simulink model "Seyfi_Ahmadi_Project4"  (R2018b)
settings: Solver=VariableStepAuto  StartTime=0.0  StopTime=50  RelTol=1e-3
settings Model: Creator=DearUser  LastModifiedBy=DearUser

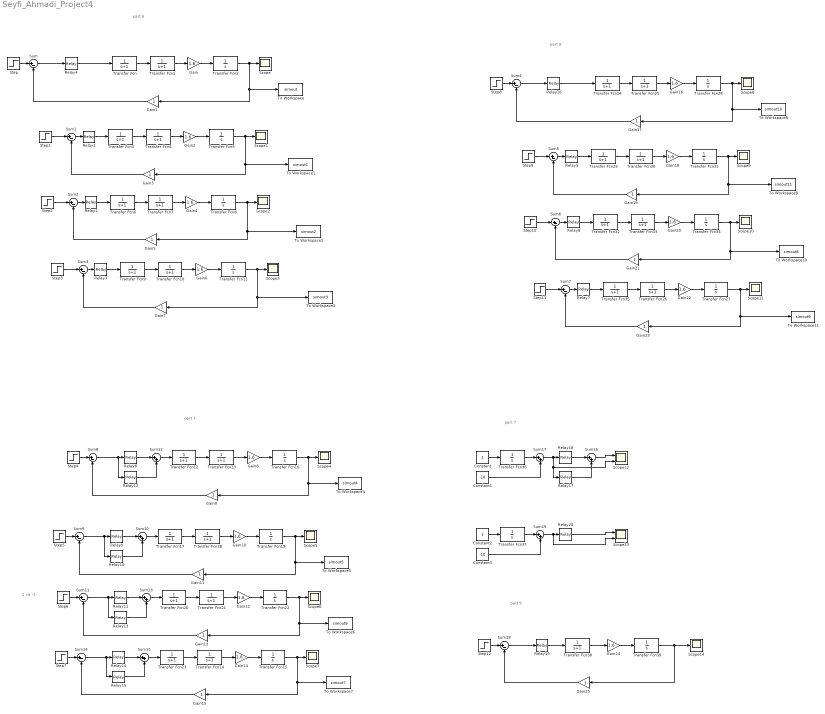
== system Seyfi_Ahmadi_Project4 ==
  note: 1 va -1
  note: part 6
  note: part 7
  note: part 8
  note: part 7
  note: part 9
  Constant : Constant
  Constant1 : Constant  Value=-10
  Constant2 : Constant
  Constant3 : Constant  Value=-10
  Gain{,2,4,6,8,10,12,14,16,18,20,22,24} (13 alike) : Gain  Gain=1.6
  Gain{1,3,5,7,9,11,13,15,17,19,21,23,25} (13 alike) : Gain
  Relay{1..3,7} (4 alike) : Relay  OnSwitchValue=0  OffSwitchValue=0  OnOutputValue=5  OffOutputValue=-5
  Relay10 : Relay  OnSwitchValue=-1.5  OffSwitchValue=-2  OnOutputValue=5  OffOutputValue=-5
  Relay11 : Relay  OnSwitchValue=1  OffSwitchValue=0  OnOutputValue=2.5  OffOutputValue=-2.5
  Relay12 : Relay  OnSwitchValue=0  OffSwitchValue=0  OnOutputValue=2.5  OffOutputValue=-2.5
  Relay13 : Relay  OnSwitchValue=-1  OffSwitchValue=-2.5  OnOutputValue=2.5  OffOutputValue=-2.5
  Relay14 : Relay  OnSwitchValue=2.5  OffSwitchValue=0  OnOutputValue=2.5  OffOutputValue=-2.5
  Relay15 : Relay  OnSwitchValue=-2.5  OffSwitchValue=-4  OnOutputValue=2.5  OffOutputValue=-2.5
  Relay16 : Relay  OnSwitchValue=5  OffSwitchValue=-5  OnOutputValue=3  OffOutputValue=-3
  Relay17 : Relay  OnSwitchValue=-1.5  OffSwitchValue=-3  OnOutputValue=2.5  OffOutputValue=-2.5
  Relay18 : Relay  OnSwitchValue=1.5  OffSwitchValue=0  OnOutputValue=2.5  OffOutputValue=-2.5
  Relay19 : Relay  OnSwitchValue=5  OffSwitchValue=-5  OnOutputValue=5  OffOutputValue=-5
  Relay20 : Relay  OnSwitchValue=0  OffSwitchValue=0  OnOutputValue=2.5  OffOutputValue=-2.5
  Relay4 : Relay  OnSwitchValue=1  OffSwitchValue=-1  OnOutputValue=5  OffOutputValue=-5
  Relay5 : Relay  OnSwitchValue=5  OffSwitchValue=-5  OnOutputValue=5  OffOutputValue=-5
  Relay6 : Relay  OnSwitchValue=5  OffSwitchValue=-5  OnOutputValue=7  OffOutputValue=-7
  Relay8 : Relay  OnSwitchValue=0  OffSwitchValue=0  OnOutputValue=2.5  OffOutputValue=-2.5
  Relay9 : Relay  OnSwitchValue=1.5  OffSwitchValue=0  OnOutputValue=5  OffOutputValue=-5
  Scope{,1..11,14} (13 alike) : Scope
  Scope12 : Scope  NumInputPorts=2
  Scope13 : Scope  NumInputPorts=2
  Step : Step  Before=1  After=-1  SampleTime=0
  Step{1,4..11} (9 alike) : Step  Before=1  After=0  SampleTime=0
  Step12 : Step  Before=1  After=-1  SampleTime=0
  Step2 : Step  Before=1  SampleTime=0
  Step3 : Step  Before=1  After=2  SampleTime=0
  Sum{,1..9,11,14,18} (13 alike) : Sum  Inputs=|+-
  Sum{10,12..13,15..17,19} (7 alike) : Sum  Inputs=|++
  To Workspace : ToWorkspace  VariableName=simout  SaveFormat=Timeseries  SampleTime=-1
  To Workspace1 : ToWorkspace  VariableName=simout1  SaveFormat=Timeseries  SampleTime=-1
  To Workspace10 : ToWorkspace  VariableName=simout8  SaveFormat=Timeseries  SampleTime=-1
  To Workspace11 : ToWorkspace  VariableName=simout9  SaveFormat=Timeseries  SampleTime=-1
  To Workspace2 : ToWorkspace  VariableName=simout2  SaveFormat=Timeseries  SampleTime=-1
  To Workspace3 : ToWorkspace  VariableName=simout3  SaveFormat=Timeseries  SampleTime=-1
  To Workspace4 : ToWorkspace  VariableName=simout4  SaveFormat=Timeseries  SampleTime=-1
  To Workspace5 : ToWorkspace  VariableName=simout5  SaveFormat=Timeseries  SampleTime=-1
  To Workspace6 : ToWorkspace  VariableName=simout6  SaveFormat=Timeseries  SampleTime=-1
  To Workspace7 : ToWorkspace  VariableName=simout7  SaveFormat=Timeseries  SampleTime=-1
  To Workspace8 : ToWorkspace  VariableName=simout10  SaveFormat=Timeseries  SampleTime=-1
  To Workspace9 : ToWorkspace  VariableName=simout11  SaveFormat=Timeseries  SampleTime=-1
  Transfer Fcn{,1,3..4,6..7,9..10,12..14,17..18,20..21,23..26,29..30,32..33,35,38} (25 alike) : TransferFcn  Denominator=[1 1]
  Transfer Fcn{2,5,8,11,15..16,19,22,27..28,31,34,36..37,39} (15 alike) : TransferFcn  Denominator=[1 0]
  wires:
  Step/1 -> Sum/1
  Transfer Fcn/1 -> Transfer Fcn1/1
  Transfer Fcn1/1 -> Gain/1
  Gain/1 -> Transfer Fcn2/1
  Transfer Fcn2/1 -> To Workspace/1, Gain1/1, Scope/1
  Gain1/1 -> Sum/2
  Gain3/1 -> Sum1/2
  Transfer Fcn4/1 -> Gain2/1
  Gain2/1 -> Transfer Fcn5/1
  Transfer Fcn3/1 -> Transfer Fcn4/1
  Step1/1 -> Sum1/1
  Relay1/1 -> Transfer Fcn3/1
  Sum1/1 -> Relay1/1
  Gain5/1 -> Sum2/2
  Transfer Fcn7/1 -> Gain4/1
  Gain4/1 -> Transfer Fcn8/1
  Transfer Fcn6/1 -> Transfer Fcn7/1
  Step2/1 -> Sum2/1
  Relay2/1 -> Transfer Fcn6/1
  Sum2/1 -> Relay2/1
  Gain7/1 -> Sum3/2
  Transfer Fcn10/1 -> Gain6/1
  Gain6/1 -> Transfer Fcn11/1
  Transfer Fcn9/1 -> Transfer Fcn10/1
  Step3/1 -> Sum3/1
  Relay3/1 -> Transfer Fcn9/1
  Sum3/1 -> Relay3/1
  Transfer Fcn5/1 -> To Workspace1/1, Gain3/1, Scope1/1
  Transfer Fcn8/1 -> To Workspace2/1, Gain5/1, Scope2/1
  Transfer Fcn11/1 -> To Workspace3/1, Gain7/1, Scope3/1
  Relay4/1 -> Transfer Fcn/1
  Transfer Fcn22/1 -> To Workspace6/1, Gain13/1, Scope6/1
  Gain8/1 -> Transfer Fcn16/1
  Sum10/1 -> Transfer Fcn17/1
  Relay9/1 -> Sum10/1
  Transfer Fcn19/1 -> To Workspace5/1, Gain11/1, Scope5/1
  Step5/1 -> Sum9/1
  Sum9/1 -> Relay10/1, Relay9/1
  Transfer Fcn18/1 -> Gain10/1
  Transfer Fcn14/1 -> Gain14/1
  Sum8/1 -> Relay12/1, Relay8/1
  Gain11/1 -> Sum9/2
  Relay10/1 -> Sum10/2
  Sum12/1 -> Transfer Fcn12/1
  Step7/1 -> Sum14/1
  Transfer Fcn21/1 -> Gain12/1
  Relay15/1 -> Sum15/2
  Relay13/1 -> Sum13/2
  Sum15/1 -> Transfer Fcn23/1
  Gain13/1 -> Sum11/2
  Transfer Fcn20/1 -> Transfer Fcn21/1
  Gain12/1 -> Transfer Fcn22/1
  Gain15/1 -> Sum14/2
  Sum11/1 -> Relay13/1, Relay11/1
  Transfer Fcn13/1 -> Gain8/1
  Step4/1 -> Sum8/1
  Gain10/1 -> Transfer Fcn19/1
  Relay11/1 -> Sum13/1
  Step6/1 -> Sum11/1
  Sum13/1 -> Transfer Fcn20/1
  Transfer Fcn12/1 -> Transfer Fcn13/1
  Gain14/1 -> Transfer Fcn15/1
  Transfer Fcn15/1 -> To Workspace7/1, Gain15/1, Scope7/1
  Sum14/1 -> Relay15/1, Relay14/1
  Transfer Fcn16/1 -> To Workspace4/1, Gain9/1, Scope4/1
  Relay12/1 -> Sum12/2
  Gain9/1 -> Sum8/2
  Relay14/1 -> Sum15/1
  Relay8/1 -> Sum12/1
  Transfer Fcn23/1 -> Transfer Fcn14/1
  Transfer Fcn17/1 -> Transfer Fcn18/1
  Sum/1 -> Relay4/1
  Gain17/1 -> Sum4/2
  Transfer Fcn28/1 -> To Workspace8/1, Gain17/1, Scope8/1
  Transfer Fcn24/1 -> Transfer Fcn25/1
  Sum4/1 -> Relay16/1
  Transfer Fcn25/1 -> Gain16/1
  Relay16/1 -> Transfer Fcn24/1
  Step8/1 -> Sum4/1
  Transfer Fcn35/1 -> Transfer Fcn26/1
  Step11/1 -> Sum7/1
  Relay7/1 -> Transfer Fcn35/1
  Transfer Fcn27/1 -> To Workspace11/1, Gain23/1, Scope11/1
  Gain23/1 -> Sum7/2
  Transfer Fcn26/1 -> Gain22/1
  Step10/1 -> Sum6/1
  Sum6/1 -> Relay6/1
  Relay6/1 -> Transfer Fcn32/1
  Transfer Fcn33/1 -> Gain20/1
  Gain16/1 -> Transfer Fcn28/1
  Gain21/1 -> Sum6/2
  Gain19/1 -> Sum5/2
  Gain22/1 -> Transfer Fcn27/1
  Sum5/1 -> Relay5/1
  Gain20/1 -> Transfer Fcn34/1
  Sum7/1 -> Relay7/1
  Transfer Fcn31/1 -> To Workspace9/1, Gain19/1, Scope9/1
  Relay5/1 -> Transfer Fcn29/1
  Transfer Fcn34/1 -> To Workspace10/1, Gain21/1, Scope10/1
  Transfer Fcn30/1 -> Gain18/1
  Transfer Fcn29/1 -> Transfer Fcn30/1
  Gain18/1 -> Transfer Fcn31/1
  Transfer Fcn32/1 -> Transfer Fcn33/1
  Step9/1 -> Sum5/1
  Constant/1 -> Transfer Fcn36/1
  Relay17/1 -> Sum16/2
  Relay18/1 -> Sum16/1
  Sum16/1 -> Scope12/1
  Transfer Fcn36/1 -> Sum17/1
  Sum17/1 -> Relay17/1, Scope12/2, Relay18/1
  Constant1/1 -> Sum17/2
  Constant2/1 -> Transfer Fcn37/1
  Constant3/1 -> Sum19/2
  Transfer Fcn37/1 -> Sum19/1
  Relay20/1 -> Scope13/1
  Sum19/1 -> Scope13/2, Relay20/1
  Sum18/1 -> Relay19/1
  Step12/1 -> Sum18/1
  Transfer Fcn38/1 -> Gain24/1
  Gain24/1 -> Transfer Fcn39/1
  Transfer Fcn39/1 -> Gain25/1, Scope14/1
  Gain25/1 -> Sum18/2
  Relay19/1 -> Transfer Fcn38/1
